simulink library "abc_dq_lib_2011"  (Simulink 7.8)
settings: Solver=ode45  StartTime=0.0  StopTime=10.0  RelTol=1e-3
settings Model: Creator=CH24070  LastModifiedBy=CH24070

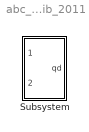
== system abc_dq_lib_2011 ==
  Subsystem : Subsystem

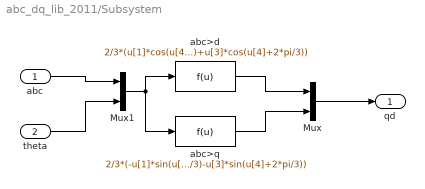
== system abc_dq_lib_2011/Subsystem ==
  abc : Inport  OutDataTypeStr=double  PortDimensions=3
  theta : Inport  Port=2  OutDataTypeStr=double  PortDimensions=1
  Mux : Mux  Inputs=2
  Mux1 : Mux  Inputs=2
  abc>d : Fcn  Expr=2/3*(u[1]*cos(u[4])+u[2]*cos(u[4]-2*pi/3)+u[3]*cos(u[4]+2*pi/3))
  abc>q : Fcn  Expr=2/3*(-u[1]*sin(u[4])-u[2]*sin(u[4]-2*pi/3)-u[3]*sin(u[4]+2*pi/3))
  qd : Outport  OutDataTypeStr=double  PortDimensions=2
  wires:
  Mux1/1 -> abc>q/1, abc>d/1
  Mux/1 -> qd/1
  abc>d/1 -> Mux/1
  abc>q/1 -> Mux/2
  theta/1 -> Mux1/2
  abc/1 -> Mux1/1
